simulink model "DOUBLE_pendulum"  (R2019b)
settings: Solver=ode45  StartTime=0  StopTime=25  FixedStep=1e-8  MaxStep=.01  RelTol=1e-6  AbsTol=1e-8  EnableMultiTasking=on
InitFcn:
  | m1=10; m2=m1;
  | L1=5; L2=L1;
  | g=9.8;
  | K1=1/(L1*(m1+m2));
  | K2=(m1+m2)*g;
  | K3=m2*L2;
  | K4=m2*L2;
  | K5=m2*L1;
  | K6=1/(m2*L2);
  | K7=m2*g;
settings Model: Creator=David  LastModifiedBy=sulaymon.eshkabilov
settings SolverCC: AutoScaleAbsTol=off  AutoInsertRateTranBlk=on
settings OptimizationCC: ExpressionDepthLimit=2147483647  LifeSpan=inf
settings DebuggingCC: UnderspecifiedInitializationDetection=Classic  MergeDetectMultiDrivingBlocksExec=none  SolverPrmCheckMsg=warning  StateNameClashWarn=warning  SFUnexpectedBacktrackingDiag=warning  SFNoUnconditionalDefaultTransitionDiag=warning  SFExecutionAtInitializationDiag=none  ArithmeticOperatorsInVariantConditions=warning
settings HardwareCC: ProdBitPerPointer=32  ProdBitPerSizeT=32  ProdBitPerPtrDiffT=32  ProdLargestAtomicFloat=None  ProdIntDivRoundTo=Undefined  ProdEndianess=Unspecified  ProdWordSize=32  ProdHWDeviceType=32-bit Generic
settings ModelReferenceCC: PropagateSignalLabelsOutOfModel=off
settings SFSimCC: SimUseLocalCustomCode=off  CustomCodeUndefinedFunction=UseInterfaceOnly
settings RTWCC: RTWUseLocalCustomCode=off
settings CodeAppCC: StateflowObjectComments=on
settings GRTTargetCC: TargetLangStandard=C89/C90 (ANSI)  GeneratePreprocessorConditionals=Disable all
settings ConfigComp: CovMetricSettings=dw  CovHtmlReporting=on  CovSaveCumulativeToWorkspaceVar=on  CovSaveSingleToWorkspaceVar=on  CovExternalEMLEnable=off

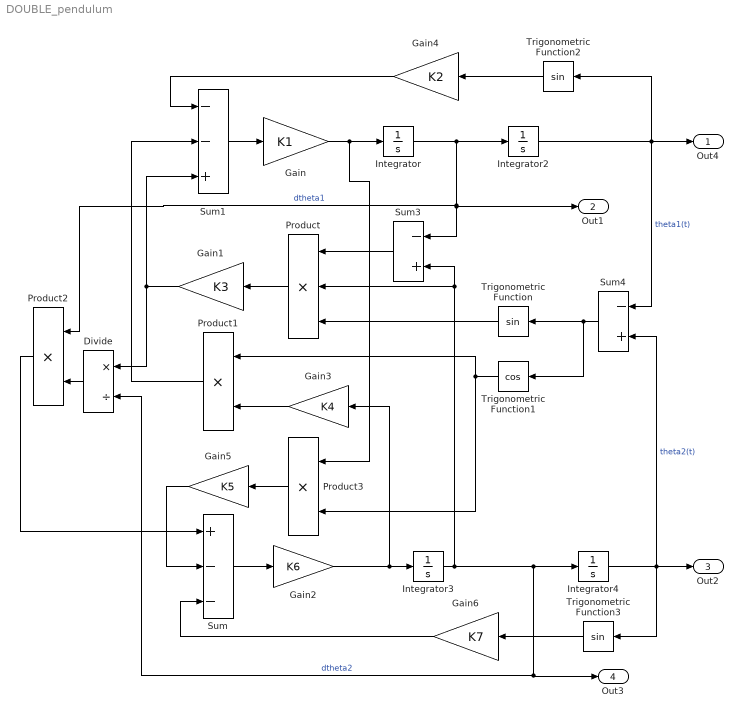
== system DOUBLE_pendulum ==
  Divide : Product  Inputs=*/
  Gain : Gain  Gain=K1
  Gain1 : Gain  Gain=K3
  Gain2 : Gain  Gain=K6
  Gain3 : Gain  Gain=K4
  Gain4 : Gain  Gain=K2
  Gain5 : Gain  Gain=K5
  Gain6 : Gain  Gain=K7
  Integrator : Integrator  InitialCondition=-1
  Integrator2 : Integrator  InitialCondition=-0.5
  Integrator3 : Integrator  InitialCondition=2
  Integrator4 : Integrator  InitialCondition=1
  Product : Product  Inputs=3  RndMeth=Zero
  Product1 : Product  RndMeth=Zero
  Product2 : Product  RndMeth=Ceiling
  Product3 : Product  RndMeth=Ceiling
  Sum : Sum  RequirementInfo={} %GIDa_5108bf6c_5f1d_4661_9113_481c46f0b7b4  Inputs=+--
  Sum1 : Sum  Inputs=--+
  Sum3 : Sum  Inputs=-+
  Sum4 : Sum  Inputs=-+
  Trigonometric Function : Trigonometry
  Trigonometric Function1 : Trigonometry  Operator=cos
  Trigonometric Function2 : Trigonometry
  Trigonometric Function3 : Trigonometry
  Out4 : Outport
  Out1 : Outport  Port=2
  Out2 : Outport  Port=3
  Out3 : Outport  Port=4
  wires:
  Gain/1 -> Product3/1, Integrator/1
  Integrator2/1 -> Out4/1, Trigonometric Function2/1, Sum4/1  "theta1(t)"
  Gain2/1 -> Integrator3/1, Gain3/1
  Integrator4/1 -> Out2/1, Trigonometric Function3/1, Sum4/2  "theta2(t)"
  Sum1/1 -> Gain/1
  Sum/1 -> Gain2/1
  Sum3/1 -> Product/1
  Sum4/1 -> Trigonometric Function1/1, Trigonometric Function/1
  Product/1 -> Gain1/1
  Trigonometric Function/1 -> Product/3
  Trigonometric Function1/1 -> Product3/2, Product1/1
  Gain3/1 -> Product1/2
  Product1/1 -> Sum1/2
  Trigonometric Function2/1 -> Gain4/1
  Gain4/1 -> Sum1/1
  Gain1/1 -> Sum1/3, Divide/1
  Product3/1 -> Gain5/1
  Gain5/1 -> Sum/2
  Trigonometric Function3/1 -> Gain6/1
  Gain6/1 -> Sum/3
  Integrator/1 -> Integrator2/1, Product2/1, Out1/1, Sum3/1  "dtheta1"
  Integrator3/1 -> Out3/1, Divide/2, Integrator4/1, Product/2, Sum3/2  "dtheta2"
  Product2/1 -> Sum/1
  Divide/1 -> Product2/2
